simulink model "PembahasanTugasElinTrainSim"  (R2021a)
settings: Solver=VariableStepAuto  StartTime=0.0  StopTime=1000  RelTol=1e-3
settings Model: Creator=asus  LastModifiedBy=asus

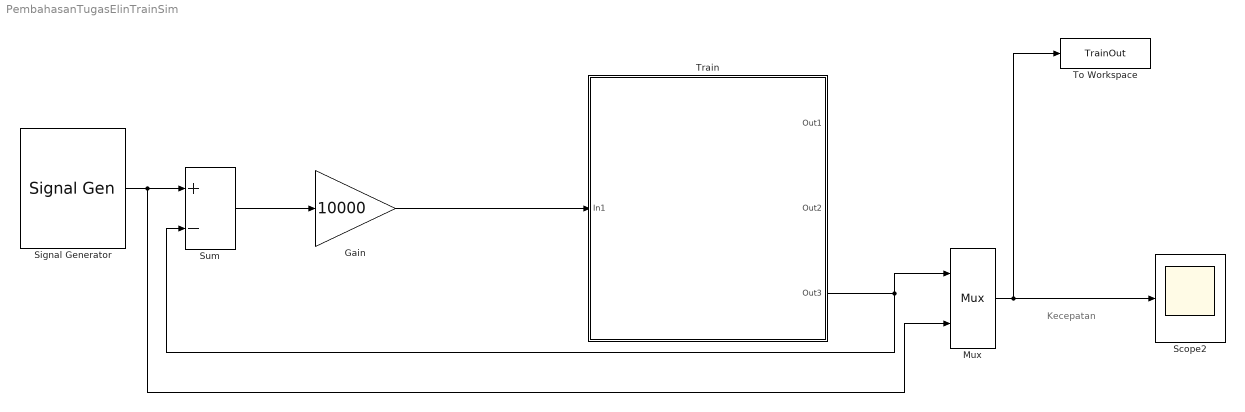
== system PembahasanTugasElinTrainSim ==
  note: Kecepatan
  Gain : Gain  Gain=10000
  Mux : Mux  Inputs=2
  Scope2 : Scope
  Signal Generator : SignalGenerator  WaveForm=square  Amplitude=-1  Frequency=0.001
  Sum : Sum  Inputs=+-
  To Workspace : ToWorkspace  VariableName=TrainOut  SaveFormat=Timeseries  SampleTime=-1
  Train : Subsystem  mask(Sistem Kereta Api){M1=1, M2=0.5, k=1, mu=0.02, g=10, F=1}
      mask prompts: M1 "Massa1(kg)"; M2 "Massa2(kg)"; k "konstanta pegas(N/m)"; mu "koefisien gesek(Ns)"; g "percepatan gravitasi(M/s^2)"; F "gaya mesin(N)"
      mask help: Silakan masukan nilai paramter system berikut
      mask init:
      | M1 > 0
      | M2 > 0
      | k > 0
      | mu > 0
      | g > 0
      | F > 0
      mask Display: image("C:\Users\asus\Downloads\pngtree-cartoon-train-illustration-png-image_8780793.png")
  wires:
  Train/3(Out3) -> Mux/1, Sum/2
  Gain/1 -> Train/1(In1)
  Sum/1 -> Gain/1
  Signal Generator/1 -> Mux/2, Sum/1
  Mux/1 -> Scope2/1, To Workspace/1

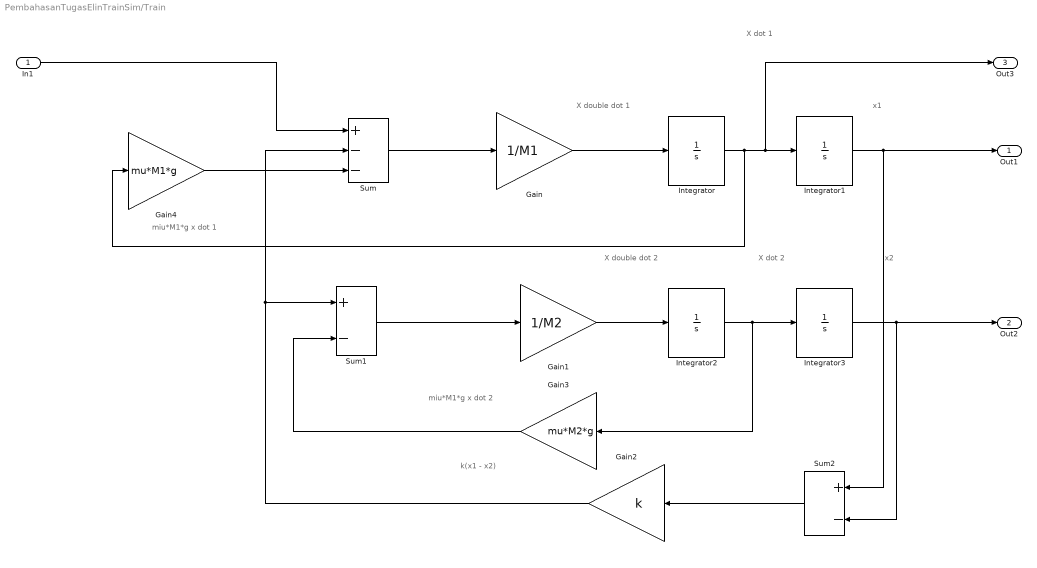
== system PembahasanTugasElinTrainSim/Train ==
  note: X double dot 1
  note: X dot 1
  note: x1
  note: x2
  note: X double dot 2
  note: X dot 2
  note: miu*M1*g x dot 1
  note: k(x1 - x2)
  note: miu*M1*g x dot 2
  In1 : Inport
  Gain : Gain  Gain=1/M1
  Gain1 : Gain  Gain=1/M2
  Gain2 : Gain  Gain=k
  Gain3 : Gain  Gain=mu*M2*g
  Gain4 : Gain  Gain=mu*M1*g
  Integrator{,1..3} (4 alike) : Integrator
  Sum : Sum  Inputs=+--
  Sum1 : Sum  Inputs=+-
  Sum2 : Sum  Inputs=+-
  Out1 : Outport
  Out2 : Outport  Port=2
  Out3 : Outport  Port=3
  wires:
  Integrator2/1 -> Gain3/1, Integrator3/1
  Sum/1 -> Gain/1
  Gain/1 -> Integrator/1
  Integrator/1 -> Integrator1/1, Out3/1, Gain4/1
  Sum2/1 -> Gain2/1
  Gain4/1 -> Sum/3
  Gain1/1 -> Integrator2/1
  Integrator1/1 -> Out1/1, Sum2/1
  Integrator3/1 -> Out2/1, Sum2/2
  Sum1/1 -> Gain1/1
  Gain3/1 -> Sum1/2
  In1/1 -> Sum/1
  Gain2/1 -> Sum/2, Sum1/1
